simulink model "lab06q2"  (Simulink 7.1)
settings: Solver=ode45  StartTime=0.0  StopTime=100  RelTol=1e-3
InitFcn:
  | RC = 2;
  | K= 1;
  | 
  | 
  | A = [(-1/RC)*(2-K) (1/RC)*K (-1/RC);(1/RC)*K (1/RC)*K (-1/RC);(1/(2*RC))*(1+2*K) (1/(2*RC))*(1+2*K) (-1/RC)]
  | 
  | B = [(1/RC)*(2-K);(-1/RC)*K;(-1/RC)*K]
  | 
  | C = [-(1+K) -(1+K) 0;1 0 0;0 1 0;0 0 1]
  | 
  | D = [(1+K);0;0;0]
libraries: simulink x7
settings Model: Creator=ALUNO  LastModifiedBy=ALUNO

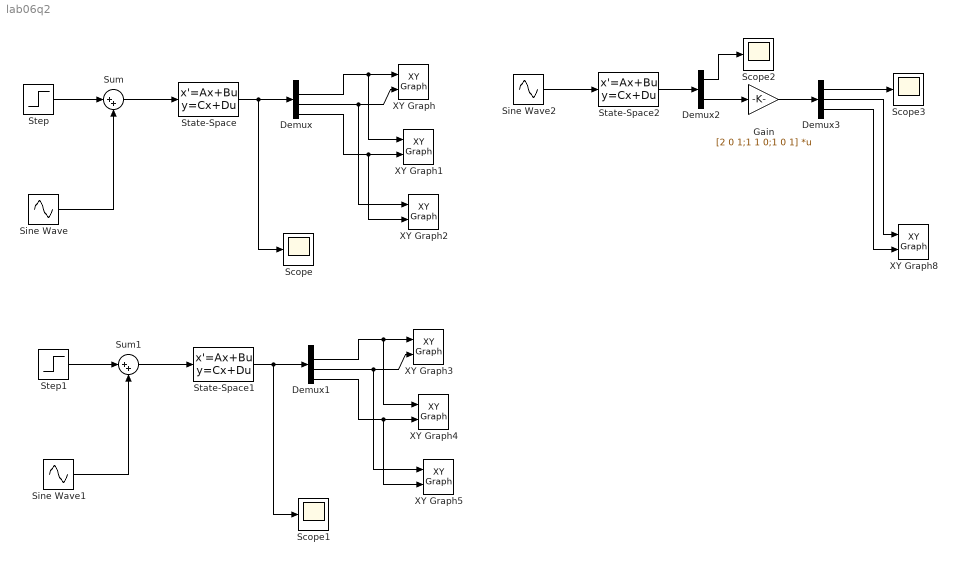
== system lab06q2 ==
  Demux : Demux
  Demux1 : Demux
  Demux2 : Demux  Outputs=[1 3]
  Demux3 : Demux  Outputs=3
  Gain : Gain  Gain=[2 0 1;1 1 0;1 0 1]  Multiplication=Matrix(K*u) (u vector)  ParameterDataType=sfix(16)  ParameterScaling=2^0  OutDataType=sfix(16)  OutScaling=2^0
  Scope{,1..3} (4 alike) : Scope
      Scope2 settings: SaveName=ScopeData2
      Scope3 settings: SaveName=ScopeData3
  Sine Wave : Sin  Frequency=5  SampleTime=0
  Sine Wave1 : Sin  Frequency=0.5  SampleTime=0
  Sine Wave2 : Sin  Frequency=5  SampleTime=0
  State-Space : StateSpace  A=A  B=B  C=C  D=D
  State-Space1 : StateSpace  A=A  B=B  C=C  D=D
  State-Space2 : StateSpace  A=A  B=B  C=C  D=D
  Step : Step  Time=0  Before=1  SampleTime=0
  Step1 : Step  Time=0  Before=1  SampleTime=0
  Sum : Sum  Inputs=|++  OutDataType=sfix(16)  OutScaling=2^0
  Sum1 : Sum  Inputs=|++  OutDataType=sfix(16)  OutScaling=2^0
  XY Graph{,1..5,8} (7 alike) : simulink/Sinks/XY Graph  SystemSampleTime=-1  xmin=-2  xmax=2  ymin=-2  ymax=2  st=-1
  wires:
  Step/1 -> Sum/1
  Sine Wave/1 -> Sum/2
  Sum/1 -> State-Space/1
  State-Space/1 -> Demux/1, Scope/1
  Demux/2 -> XY Graph/1, XY Graph1/1
  Demux/3 -> XY Graph/2, XY Graph2/1
  Demux/4 -> XY Graph1/2, XY Graph2/2
  Step1/1 -> Sum1/1
  Sine Wave1/1 -> Sum1/2
  Sum1/1 -> State-Space1/1
  State-Space1/1 -> Demux1/1, Scope1/1
  Demux1/2 -> XY Graph3/1, XY Graph4/1
  Demux1/3 -> XY Graph3/2, XY Graph5/1
  Demux1/4 -> XY Graph4/2, XY Graph5/2
  Sine Wave2/1 -> State-Space2/1
  State-Space2/1 -> Demux2/1
  Demux2/2 -> Gain/1
  Gain/1 -> Demux3/1
  Demux2/1 -> Scope2/1
  Demux3/1 -> Scope3/1
  Demux3/2 -> XY Graph8/1
  Demux3/3 -> XY Graph8/2
